simulink model "ACC_final_ver_2"  (R2021b)
settings: Solver=FixedStepAuto  StartTime=0.0  StopTime=inf  FixedStep=0.01  RelTol=1e-3  EnableMultiTasking=on
libraries: arduinolib x6, arduinosensorlib x3
settings Model: ExtModeTrigDuration=2  Creator=user  LastModifiedBy=user
settings OptimizationCC: EnhancedBackFolding=on  PassReuseOutputArgsAs=Individual arguments  ZeroExternalMemoryAtStartup=off  ZeroInternalMemoryAtStartup=off  MaxStackSize=64  OptimizeBlockOrder=speed  DifferentSizesBufferReuse=on  OptimizationCustomize=off  EfficientTunableParamExpr=on
settings DebuggingCC: MultiTaskDSMMsg=none  ParameterTunabilityLossMsg=error
settings HardwareCC: ProdBitPerInt=16  ProdBitPerPointer=16  ProdBitPerSizeT=16  ProdBitPerPtrDiffT=16  ProdLargestAtomicFloat=None  ProdWordSize=8  ProdHWDeviceType=Atmel->AVR
settings SFSimCC: MATLABDynamicMemAlloc=off
settings RTWCC: Description=Embedded Coder  SystemTargetFile=ert.tlc  HardwareBoard=Arduino Mega 2560  TemplateMakefile=ert_default_tmf  Toolchain=Arduino AVR  BuildConfiguration=Faster Runs
settings CodeAppCC: ForceParamTrailComments=on  IgnoreCustomStorageClasses=off  OperatorAnnotations=on  SimulinkDataObjDesc=on  SFDataObjDesc=on  InsertBlockDesc=on
settings ERTTargetCC: SupportContinuousTime=on  SupportVariableSizeSignals=on  ExtModeTransport=3  ExtModeStaticAlloc=on  ExtModeStaticAllocSize=2048  ExtModeMexFile=ext_xcp  ExtModeIntrfLevel=Level2 - Open

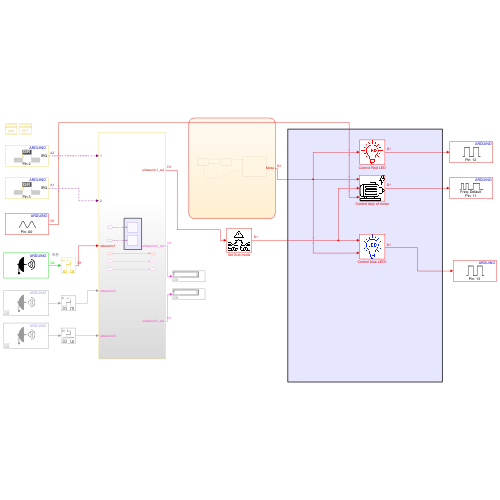
[thumbnail: Simulink's stored preview of the top-level diagram]
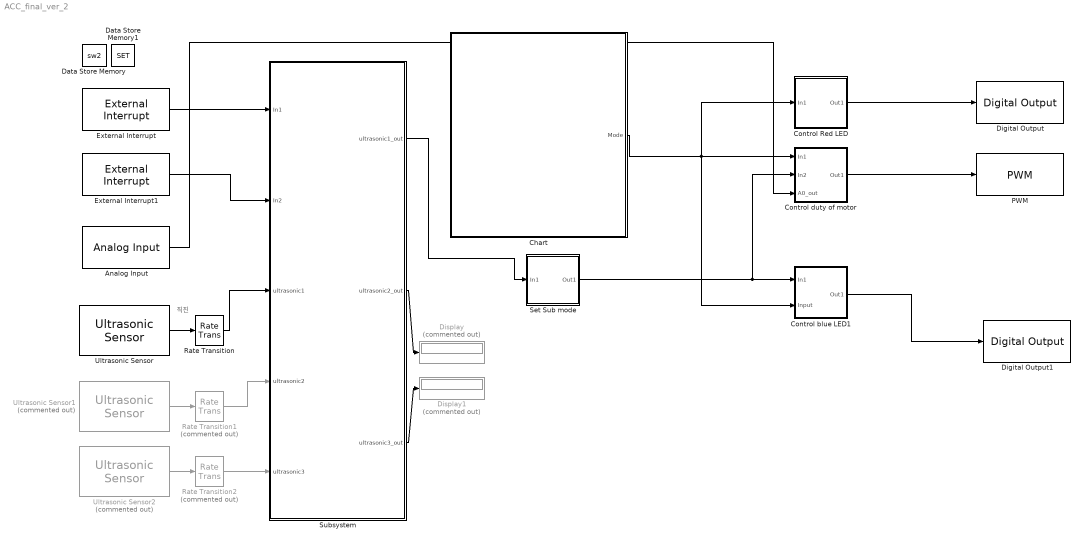
== system ACC_final_ver_2 ==
  note: 직진
  Analog Input : arduinolib/Analog Input  pinNumber=0  ReadResultsOnly=off  ConversionTriggerSource=Software  ExternalTriggerType=uint32( 0 )  OutputDataType=uint16  EnableConversionCompleteNotify=off  EnableOuputStatus=off  SampleTime=-1  blockPlatform=arduino
  Chart : Stateflow chart  TreatAsAtomicUnit=on
  Control Red LED : Subsystem
      mask Display: image('$imagefile'); % 변경하려면 툴스트립에 있는 "이미지 편집"을 사용하십시오.
  Control blue LED1 : Subsystem
      mask Display: image('$imagefile'); % 변경하려면 툴스트립에 있는 "이미지 편집"을 사용하십시오.
  Control duty of motor : Subsystem
      mask Display: image('$imagefile'); % 변경하려면 툴스트립에 있는 "이미지 편집"을 사용하십시오.
  Data Store Memory : DataStoreMemory  DataStoreName=sw2  ReadBeforeWriteMsg=warning  WriteAfterWriteMsg=warning  WriteAfterReadMsg=warning  InitialValue=1  ShareAcrossModelInstances=on  ShowAdditionalParam=off  OutDataTypeStr=double
  Data Store Memory1 : DataStoreMemory  DataStoreName=SET  ReadBeforeWriteMsg=warning  WriteAfterWriteMsg=warning  WriteAfterReadMsg=warning  ShareAcrossModelInstances=on  ShowAdditionalParam=off  OutDataTypeStr=int8
      settings: LockScale=on
  Digital Output : arduinolib/Digital Output  pinNumber=12  Direction=output  blockPlatform=arduino
  Digital Output1 : arduinolib/Digital Output  pinNumber=13  Direction=output  blockPlatform=arduino
  Display : Display  Commented=on
  Display1 : Display  Commented=on
  External Interrupt : arduinolib/External Interrupt  Pin=2  PullUp=on  Mode=FALLING  InterruptSimulationInput=off
      settings: SourceProductBaseCode=ARDUINO
  External Interrupt1 : arduinolib/External Interrupt  Pin=3  PullUp=on  Mode=FALLING  InterruptSimulationInput=off
      settings: SourceProductBaseCode=ARDUINO
  PWM : arduinolib/PWM  pinNumber=11  frequencyType=Default  desiredFrequency=490.2  achievableFrequency=490.2
  Rate Transition : RateTransition  Deterministic=off  OutPortSampleTime=0.01
  Rate Transition1 : RateTransition  Commented=on  Deterministic=off  OutPortSampleTime=0.01
  Rate Transition2 : RateTransition  Commented=on  Deterministic=off  OutPortSampleTime=0.01
  Set Sub mode : Subsystem
      mask Display: image('$imagefile'); % 변경하려면 툴스트립에 있는 "이미지 편집"을 사용하십시오.
  Subsystem : Subsystem
  Ultrasonic Sensor : arduinosensorlib/Ultrasonic Sensor  NumSignalPins=2  TrigPin=50  EchoPin=51  SignalPin=3  SampleTime_=0.1  blockPlatform=ARDUINO
      settings: SourceProductBaseCode=ARDUINO
  Ultrasonic Sensor1 : arduinosensorlib/Ultrasonic Sensor  Commented=on  NumSignalPins=2  TrigPin=48  EchoPin=49  SignalPin=3  SampleTime_=0.1  blockPlatform=ARDUINO
      settings: SourceProductBaseCode=ARDUINO
  Ultrasonic Sensor2 : arduinosensorlib/Ultrasonic Sensor  Commented=on  NumSignalPins=2  TrigPin=46  EchoPin=47  SignalPin=3  SampleTime_=0.1  blockPlatform=ARDUINO
      settings: SourceProductBaseCode=ARDUINO
  wires:
  Chart/1(Mode) -> Control Red LED/1(In1), Control duty of motor/1(In1), Control blue LED1/2(Input)
  Set Sub mode/1(Out1) -> Control blue LED1/1(In1), Control duty of motor/2(In2)
  Control Red LED/1(Out1) -> Digital Output/1
  Control blue LED1/1(Out1) -> Digital Output1/1
  Control duty of motor/1(Out1) -> PWM/1
  Analog Input/1 -> Control duty of motor/3(A0_out)
  Ultrasonic Sensor/1 -> Rate Transition/1
  Subsystem/1(ultrasonic1_out) -> Set Sub mode/1(In1)
  Ultrasonic Sensor1/1 -> Rate Transition1/1
  External Interrupt/1 -> Subsystem/1(In1)
  External Interrupt1/1 -> Subsystem/2(In2)
  Rate Transition/1 -> Subsystem/3(ultrasonic1)
  Rate Transition1/1 -> Subsystem/4(ultrasonic2)
  Ultrasonic Sensor2/1 -> Rate Transition2/1
  Rate Transition2/1 -> Subsystem/5(ultrasonic3)
  Subsystem/2(ultrasonic2_out) -> Display/1
  Subsystem/3(ultrasonic3_out) -> Display1/1

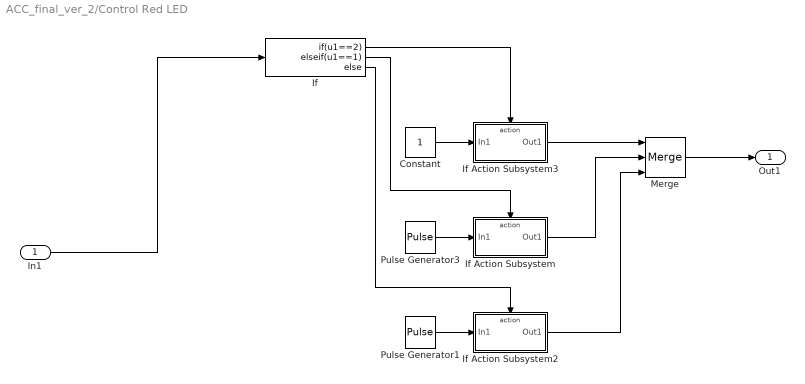
== system ACC_final_ver_2/Control Red LED ==
  In1 : Inport
  Constant : Constant
  If : If  IfExpression=u1==2  ElseIfExpressions=u1==1
  If Action Subsystem : Subsystem  TreatAsAtomicUnit=on
  If Action Subsystem2 : Subsystem  TreatAsAtomicUnit=on
  If Action Subsystem3 : Subsystem  TreatAsAtomicUnit=on
  Merge : Merge  Inputs=3
  Pulse Generator1 : DiscretePulseGenerator  Period=200  PulseWidth=100  SampleTime=-1
  Pulse Generator3 : DiscretePulseGenerator  Period=40  PulseWidth=20  SampleTime=-1
  Out1 : Outport
  wires:
  If Action Subsystem2/1(Out1) -> Merge/3
  Pulse Generator1/1 -> If Action Subsystem2/1(In1)
  Pulse Generator3/1 -> If Action Subsystem/1(In1)
  Merge/1 -> Out1/1
  If Action Subsystem/1(Out1) -> Merge/2
  If/1 -> If Action Subsystem3/Action
  If/2 -> If Action Subsystem/Action
  Constant/1 -> If Action Subsystem3/1(In1)
  If/3 -> If Action Subsystem2/Action
  If Action Subsystem3/1(Out1) -> Merge/1
  In1/1 -> If/1

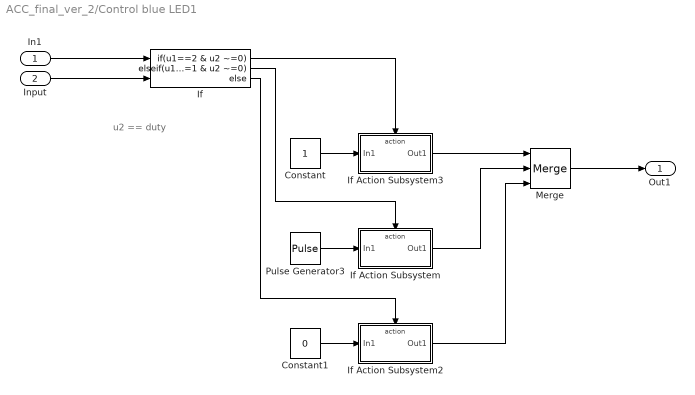
== system ACC_final_ver_2/Control blue LED1 ==
  note: u2 == duty
  In1 : Inport
  Input : Inport  Port=2
  Constant : Constant
  Constant1 : Constant  Value=0
  If : If  NumInputs=2  IfExpression=u1==2 & u2 ~=0  ElseIfExpressions=u1==1 & u2 ~=0
  If Action Subsystem : Subsystem  TreatAsAtomicUnit=on
  If Action Subsystem2 : Subsystem  TreatAsAtomicUnit=on
  If Action Subsystem3 : Subsystem  TreatAsAtomicUnit=on
  Merge : Merge  Inputs=3
  Pulse Generator3 : DiscretePulseGenerator  Period=40  PulseWidth=20  SampleTime=-1
  Out1 : Outport
  wires:
  If Action Subsystem2/1(Out1) -> Merge/3
  Constant1/1 -> If Action Subsystem2/1(In1)
  Pulse Generator3/1 -> If Action Subsystem/1(In1)
  Merge/1 -> Out1/1
  If Action Subsystem/1(Out1) -> Merge/2
  If/1 -> If Action Subsystem3/Action
  If/2 -> If Action Subsystem/Action
  Constant/1 -> If Action Subsystem3/1(In1)
  If/3 -> If Action Subsystem2/Action
  If Action Subsystem3/1(Out1) -> Merge/1
  In1/1 -> If/1
  Input/1 -> If/2

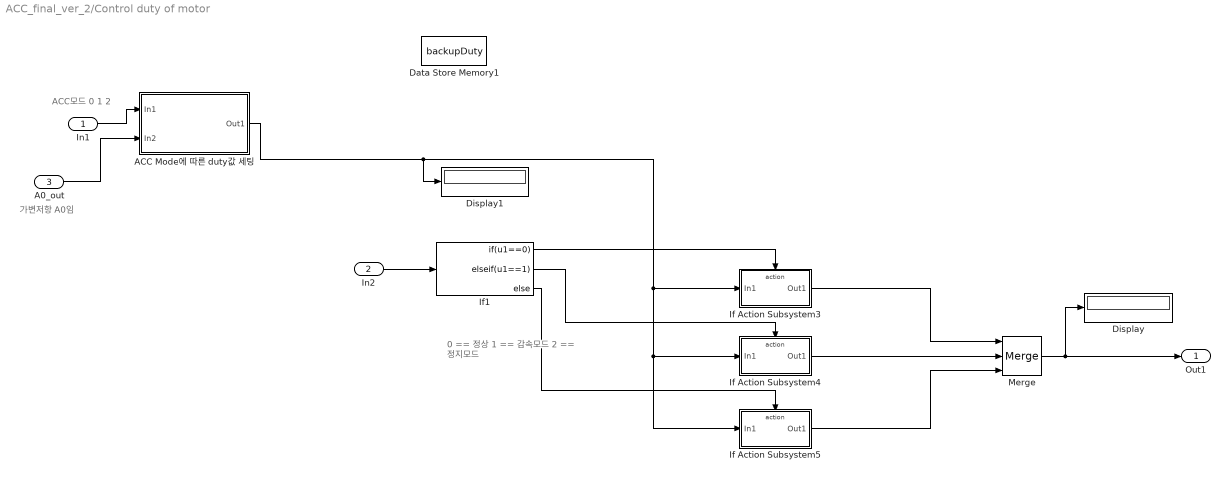
== system ACC_final_ver_2/Control duty of motor ==
  note: ACC모드 0 1 2
  note: 0 == 정상
      | 1 == 감속모드
      | 2 == 정지모드
  note: 가변저항 A0임
  In1 : Inport
  In2 : Inport  Port=2
  A0_out : Inport  Port=3
  ACC Mode에 따른 duty값 세팅 : Subsystem
  Data Store Memory1 : DataStoreMemory  DataStoreName=backupDuty  ReadBeforeWriteMsg=warning  WriteAfterWriteMsg=warning  WriteAfterReadMsg=warning  ShowAdditionalParam=off  OutDataTypeStr=uint8
  Display : Display
  Display1 : Display
  If Action Subsystem3 : Subsystem  TreatAsAtomicUnit=on
  If Action Subsystem4 : Subsystem  TreatAsAtomicUnit=on
  If Action Subsystem5 : Subsystem  TreatAsAtomicUnit=on
  If1 : If  IfExpression=u1==0  ElseIfExpressions=u1==1
  Merge : Merge  Inputs=3
  Out1 : Outport
  wires:
  In2/1 -> If1/1
  If1/2 -> If Action Subsystem4/Action
  If1/3 -> If Action Subsystem5/Action
  In1/1 -> ACC Mode에 따른 duty값 세팅/1(In1)
  ACC Mode에 따른 duty값 세팅/1(Out1) -> If Action Subsystem5/1(In1), If Action Subsystem4/1(In1), If Action Subsystem3/1(In1), Display1/1
  If1/1 -> If Action Subsystem3/Action
  If Action Subsystem3/1(Out1) -> Merge/1
  If Action Subsystem4/1(Out1) -> Merge/2
  If Action Subsystem5/1(Out1) -> Merge/3
  Merge/1 -> Out1/1, Display/1
  A0_out/1 -> ACC Mode에 따른 duty값 세팅/2(In2)

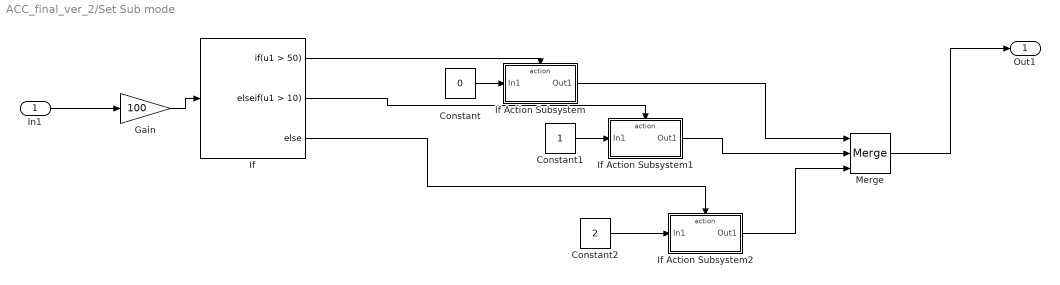
== system ACC_final_ver_2/Set Sub mode ==
  In1 : Inport
  Constant : Constant  Value=0
  Constant1 : Constant
  Constant2 : Constant  Value=2
  Gain : Gain  Gain=100
  If : If  IfExpression=u1 > 50  ElseIfExpressions=u1 > 10
  If Action Subsystem : Subsystem  TreatAsAtomicUnit=on
  If Action Subsystem1 : Subsystem  TreatAsAtomicUnit=on
  If Action Subsystem2 : Subsystem  TreatAsAtomicUnit=on
  Merge : Merge  Inputs=3
  Out1 : Outport
  wires:
  If Action Subsystem2/1(Out1) -> Merge/3
  If/2 -> If Action Subsystem1/Action
  If Action Subsystem1/1(Out1) -> Merge/2
  If Action Subsystem/1(Out1) -> Merge/1
  Gain/1 -> If/1
  Constant2/1 -> If Action Subsystem2/1(In1)
  If/1 -> If Action Subsystem/Action
  Constant1/1 -> If Action Subsystem1/1(In1)
  If/3 -> If Action Subsystem2/Action
  Constant/1 -> If Action Subsystem/1(In1)
  In1/1 -> Gain/1
  Merge/1 -> Out1/1

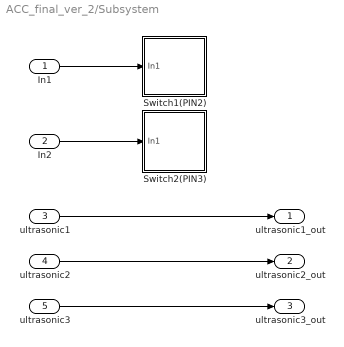
== system ACC_final_ver_2/Subsystem ==
  In1 : Inport
  In2 : Inport  Port=2
  ultrasonic1 : Inport  Port=3
  ultrasonic2 : Inport  Port=4
  ultrasonic3 : Inport  Port=5
  Switch1(PIN2) : Subsystem
      mask Display: image('$imagefile'); % 변경하려면 툴스트립에 있는 "이미지 편집"을 사용하십시오.
  Switch2(PIN3) : Subsystem
      mask Display: image('$imagefile'); % 변경하려면 툴스트립에 있는 "이미지 편집"을 사용하십시오.
  ultrasonic1_out : Outport
  ultrasonic2_out : Outport  Port=2
  ultrasonic3_out : Outport  Port=3
  wires:
  In1/1 -> Switch1(PIN2)/1(In1)
  In2/1 -> Switch2(PIN3)/1(In1)
  ultrasonic1/1 -> ultrasonic1_out/1
  ultrasonic2/1 -> ultrasonic2_out/1
  ultrasonic3/1 -> ultrasonic3_out/1

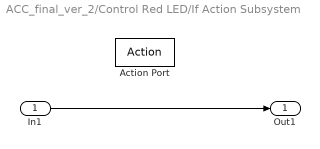
== system ACC_final_ver_2/Control Red LED/If Action Subsystem ==
  In1 : Inport
  Action Port : ActionPort  ActionPortLabel=elseif(u1==1)
  Out1 : Outport
  wires:
  In1/1 -> Out1/1

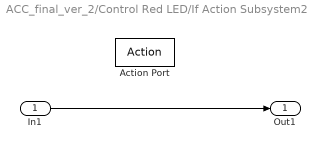
== system ACC_final_ver_2/Control Red LED/If Action Subsystem2 ==
  In1 : Inport
  Action Port : ActionPort  ActionPortLabel=else
  Out1 : Outport
  wires:
  In1/1 -> Out1/1

== system ACC_final_ver_2/Control Red LED/If Action Subsystem3 ==
  In1 : Inport
  Action Port : ActionPort  ActionPortLabel=if(u1==2)
  Out1 : Outport
  wires:
  In1/1 -> Out1/1

== system ACC_final_ver_2/Control blue LED1/If Action Subsystem ==
  In1 : Inport
  Action Port : ActionPort  ActionPortLabel=elseif(u1==1 & u2 ~=0)
  Out1 : Outport
  wires:
  In1/1 -> Out1/1

== system ACC_final_ver_2/Control blue LED1/If Action Subsystem2 ==
  In1 : Inport
  Action Port : ActionPort  ActionPortLabel=else
  Out1 : Outport
  wires:
  In1/1 -> Out1/1

== system ACC_final_ver_2/Control blue LED1/If Action Subsystem3 ==
  In1 : Inport
  Action Port : ActionPort  ActionPortLabel=if(u1==2 & u2 ~=0)
  Out1 : Outport
  wires:
  In1/1 -> Out1/1

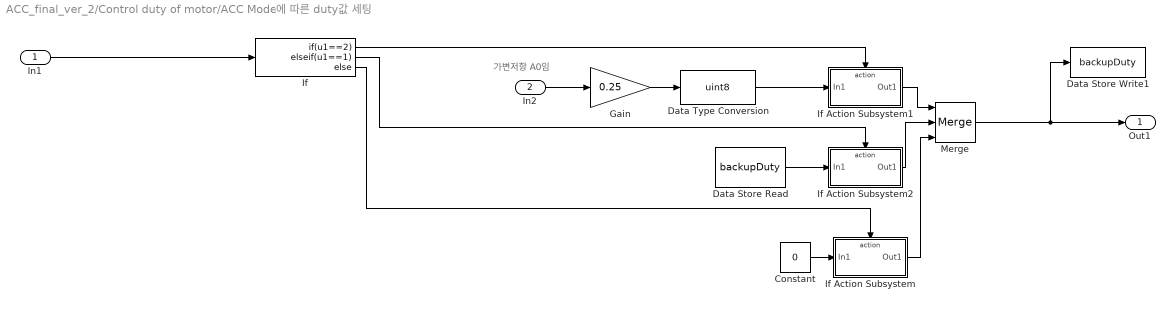
== system ACC_final_ver_2/Control duty of motor/ACC Mode에 따른 duty값 세팅 ==
  note: 가변저항 A0임
  In1 : Inport
  In2 : Inport  Port=2
  Constant : Constant  Value=0  OutDataTypeStr=uint8
  Data Store Read : DataStoreRead  DataStoreName=backupDuty  IndexOptions=Index vector (dialog)  Indices=1  OutputSizes=1
  Data Store Write1 : DataStoreWrite  DataStoreName=backupDuty  IndexOptions=Index vector (dialog)  Indices=1  OutputSizes=1
  Data Type Conversion : DataTypeConversion  OutDataTypeStr=uint8
  Gain : Gain  Gain=0.25
  If : If  IfExpression=u1==2  ElseIfExpressions=u1==1
  If Action Subsystem : Subsystem  TreatAsAtomicUnit=on
  If Action Subsystem1 : Subsystem  TreatAsAtomicUnit=on
  If Action Subsystem2 : Subsystem  TreatAsAtomicUnit=on
  Merge : Merge  Inputs=3
  Out1 : Outport
  wires:
  Constant/1 -> If Action Subsystem/1(In1)
  Data Type Conversion/1 -> If Action Subsystem1/1(In1)
  If/2 -> If Action Subsystem2/Action
  If/3 -> If Action Subsystem/Action
  Gain/1 -> Data Type Conversion/1
  Data Store Read/1 -> If Action Subsystem2/1(In1)
  Merge/1 -> Out1/1, Data Store Write1/1
  If/1 -> If Action Subsystem1/Action
  If Action Subsystem1/1(Out1) -> Merge/1
  In2/1 -> Gain/1
  If Action Subsystem2/1(Out1) -> Merge/2
  If Action Subsystem/1(Out1) -> Merge/3
  In1/1 -> If/1

== system ACC_final_ver_2/Control duty of motor/If Action Subsystem3 ==
  In1 : Inport
  Action Port : ActionPort  ActionPortLabel=if(u1==0)
  Out1 : Outport
  wires:
  In1/1 -> Out1/1

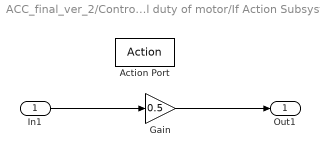
== system ACC_final_ver_2/Control duty of motor/If Action Subsystem4 ==
  In1 : Inport
  Action Port : ActionPort  ActionPortLabel=elseif(u1==1)
  Gain : Gain  Gain=0.5  OutDataTypeStr=uint8
  Out1 : Outport
  wires:
  In1/1 -> Gain/1
  Gain/1 -> Out1/1

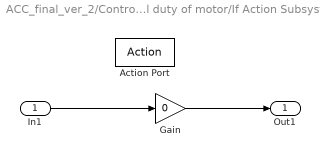
== system ACC_final_ver_2/Control duty of motor/If Action Subsystem5 ==
  In1 : Inport
  Action Port : ActionPort  ActionPortLabel=else
  Gain : Gain  Gain=0  OutDataTypeStr=uint8
  Out1 : Outport
  wires:
  In1/1 -> Gain/1
  Gain/1 -> Out1/1

== system ACC_final_ver_2/Set Sub mode/If Action Subsystem ==
  In1 : Inport
  Action Port : ActionPort  ActionPortLabel=if(u1 > 50)
  Out1 : Outport
  wires:
  In1/1 -> Out1/1

== system ACC_final_ver_2/Set Sub mode/If Action Subsystem1 ==
  In1 : Inport
  Action Port : ActionPort  ActionPortLabel=elseif(u1 > 10)
  Out1 : Outport
  wires:
  In1/1 -> Out1/1

== system ACC_final_ver_2/Set Sub mode/If Action Subsystem2 ==
  In1 : Inport
  Action Port : ActionPort  ActionPortLabel=else
  Out1 : Outport
  wires:
  In1/1 -> Out1/1

== system ACC_final_ver_2/Subsystem/Switch1(PIN2) ==
  In1 : Inport
  Function-Call Subsystem1 : Subsystem  TreatAsAtomicUnit=on
  wires:
  In1/1 -> Function-Call Subsystem1/Trigger

== system ACC_final_ver_2/Subsystem/Switch2(PIN3) ==
  In1 : Inport
  Function-Call Subsystem1 : Subsystem  TreatAsAtomicUnit=on
  wires:
  In1/1 -> Function-Call Subsystem1/Trigger

== system ACC_final_ver_2/Control duty of motor/ACC Mode에 따른 duty값 세팅/If Action Subsystem ==
  In1 : Inport
  Action Port : ActionPort  ActionPortLabel=else
  Out1 : Outport
  wires:
  In1/1 -> Out1/1

== system ACC_final_ver_2/Control duty of motor/ACC Mode에 따른 duty값 세팅/If Action Subsystem1 ==
  In1 : Inport
  Action Port : ActionPort  ActionPortLabel=if(u1==2)
  Out1 : Outport
  wires:
  In1/1 -> Out1/1

== system ACC_final_ver_2/Control duty of motor/ACC Mode에 따른 duty값 세팅/If Action Subsystem2 ==
  In1 : Inport
  Action Port : ActionPort  ActionPortLabel=elseif(u1==1)
  Out1 : Outport
  wires:
  In1/1 -> Out1/1

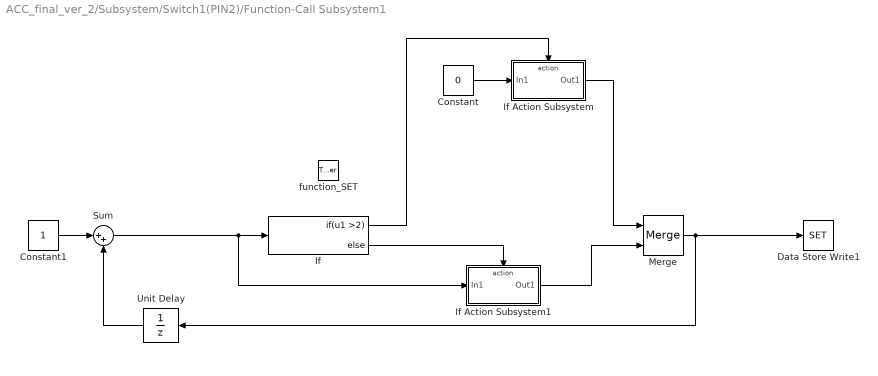
== system ACC_final_ver_2/Subsystem/Switch1(PIN2)/Function-Call Subsystem1 ==
  function_SET : TriggerPort  TriggerType=function-call  VariantControl=(inherit)
  Constant : Constant  Value=0  OutDataTypeStr=int8
  Constant1 : Constant  OutDataTypeStr=int8
  Data Store Write1 : DataStoreWrite  DataStoreName=SET  IndexOptions=Index vector (dialog)  Indices=1  OutputSizes=1
  If : If  IfExpression=u1 >2
  If Action Subsystem : Subsystem  TreatAsAtomicUnit=on
  If Action Subsystem1 : Subsystem  TreatAsAtomicUnit=on
  Merge : Merge
  Sum : Sum  Inputs=|++
  Unit Delay : UnitDelay  SampleTime=-1  HasFrameUpgradeWarning=on
  wires:
  If Action Subsystem/1(Out1) -> Merge/1
  Constant/1 -> If Action Subsystem/1(In1)
  Sum/1 -> If Action Subsystem1/1(In1), If/1
  Unit Delay/1 -> Sum/2
  If/1 -> If Action Subsystem/Action
  If/2 -> If Action Subsystem1/Action
  If Action Subsystem1/1(Out1) -> Merge/2
  Constant1/1 -> Sum/1
  Merge/1 -> Unit Delay/1, Data Store Write1/1

== system ACC_final_ver_2/Subsystem/Switch2(PIN3)/Function-Call Subsystem1 ==
  function_sw2 : TriggerPort  TriggerType=function-call  VariantControl=(inherit)
  Constant : Constant  Value=0  OutDataTypeStr=double
  Data Store Write : DataStoreWrite  DataStoreName=sw2  IndexOptions=Index vector (dialog)  Indices=1  OutputSizes=1
  wires:
  Constant/1 -> Data Store Write/1

== system ACC_final_ver_2/Subsystem/Switch1(PIN2)/Function-Call Subsystem1/If Action Subsystem ==
  In1 : Inport
  Action Port : ActionPort  ActionPortLabel=if(u1 >2)
  Out1 : Outport
  wires:
  In1/1 -> Out1/1

== system ACC_final_ver_2/Subsystem/Switch1(PIN2)/Function-Call Subsystem1/If Action Subsystem1 ==
  In1 : Inport
  Action Port : ActionPort  ActionPortLabel=else
  Out1 : Outport
  wires:
  In1/1 -> Out1/1

== stateflow chart ACC_final_ver_2/Chart ==
  state ACC_active
    Mode=2;
    %%LED_R_1s(2);
    (default) -> ? [commented out]
  state ACC_standby
    Mode=1;
    %%LED_R_1s(1);
    %speed=100;
  state ACC_off
    Mode=0;
    %%LED_R_1s(0);
  (default) -> ACC_off
  ACC_standby -> ACC_active [order 1] : [SET==2]
  ACC_off -> ACC_standby : [SET==1]
  ACC_standby -> ACC_off [order 2] : [sw2==0]{
      | sw2=1; SET=0;}
  ACC_active -> ACC_off : [SET==0||sw2==0]
  data: Mode output; sw2 data_store_memory; SET data_store_memory
